simulink subsystem "DiffSwerveChassisSimulation"  (R2022a)
settings: Solver=VariableStepAuto  StartTime=0.0  StopTime=10.0  RelTol=1e-3
values from neighbouring files (symbols this model uses):
  chassis = struct(     'M_inv', M_inv,     'M', M,     'num_modules', num_modules,     'module_locations', module_locations )    [GetDiffSwerveChassis.m]
undefined symbols (not defined in the file or in its folder): theta0, x0, y0
settings Model: Creator=woz4t  LastModifiedBy=woz4t

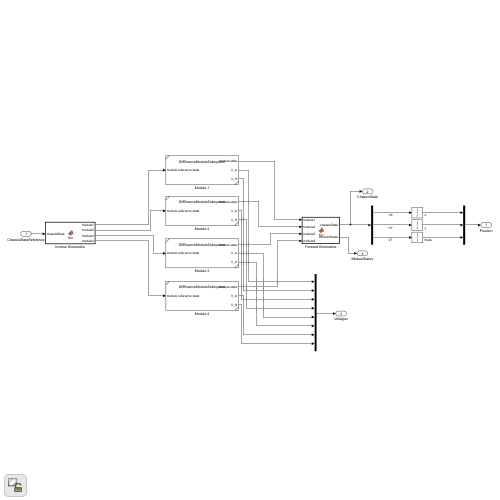
[thumbnail: Simulink's stored preview of the top-level diagram]
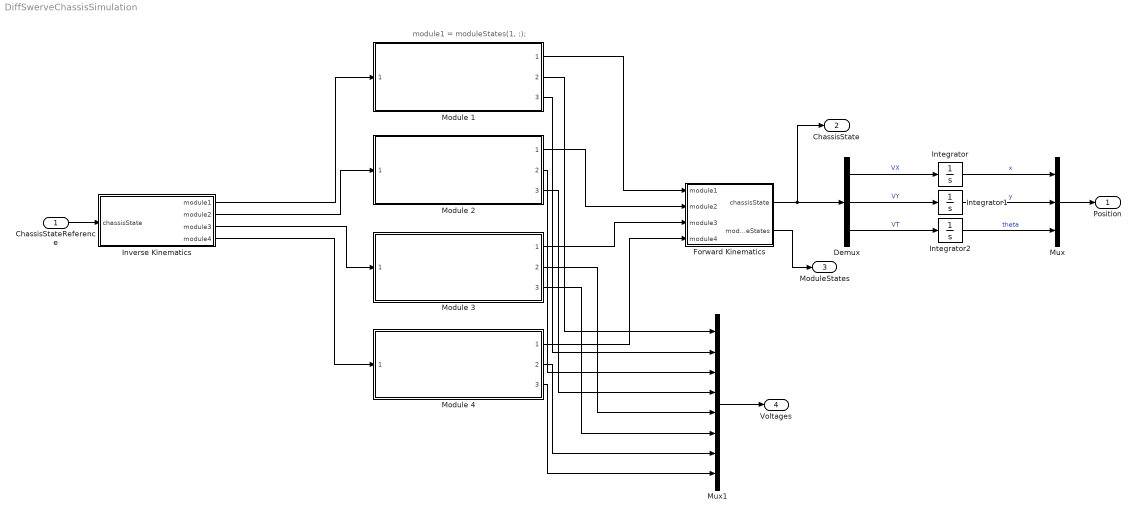
== system DiffSwerveChassisSimulation ==
  note: module1 = moduleStates(1, :);
  ChassisStateReference : Inport
  Demux : Demux  Outputs=3
  Forward Kinematics : MATLAB Function  TreatAsAtomicUnit=on  mask{M=chassis.M}
  Integrator : Integrator  InitialCondition=x0
  Integrator1 : Integrator  InitialCondition=y0
  Integrator2 : Integrator  InitialCondition=theta0
  Inverse Kinematics : MATLAB Function  TreatAsAtomicUnit=on  mask{M_inv=chassis.M_inv, num_modules=chassis.num_modules}
  Module {1..4} (4 alike) : Subsystem  ReferencedSubsystem=DiffSwerveModuleSubsystem
  Mux : Mux  Inputs=3
  Mux1 : Mux  Inputs=8
  Position : Outport
  ChassisState : Outport  Port=2
  ModuleStates : Outport  Port=3
  Voltages : Outport  Port=4
  wires:
  Integrator/1 -> Mux/1  "x"
  Forward Kinematics/1(chassisState) -> Demux/1, ChassisState/1
  Module 1/1 -> Forward Kinematics/1(module1)
  Inverse Kinematics/3(module3) -> Module 3/1
  Integrator2/1 -> Mux/3  "theta"
  Inverse Kinematics/4(module4) -> Module 4/1
  Demux/1 -> Integrator/1  "VX"
  Demux/2 -> Integrator1/1  "VY"
  ChassisStateReference/1 -> Inverse Kinematics/1(chassisState)
  Inverse Kinematics/2(module2) -> Module 2/1
  Module 3/1 -> Forward Kinematics/3(module3)
  Demux/3 -> Integrator2/1  "VT"
  Inverse Kinematics/1(module1) -> Module 1/1
  Integrator1/1 -> Mux/2  "y"
  Module 4/1 -> Forward Kinematics/4(module4)
  Module 2/1 -> Forward Kinematics/2(module2)
  Mux/1 -> Position/1
  Forward Kinematics/2(moduleStates) -> ModuleStates/1
  Module 1/2 -> Mux1/1
  Module 1/3 -> Mux1/2
  Module 2/2 -> Mux1/3
  Module 2/3 -> Mux1/4
  Module 3/2 -> Mux1/5
  Module 3/3 -> Mux1/6
  Module 4/2 -> Mux1/7
  Module 4/3 -> Mux1/8
  Mux1/1 -> Voltages/1

== matlab function DiffSwerveChassisSimulation/Forward Kinematics ==
  data: module1 input; chassisState output; module2 input; module3 input; module4 input; M parameter; moduleStates output
function [chassisState, moduleStates] = fcn(module1, module2, module3, module4, M)

moduleStates = zeros(4, 3);
moduleStates(1, :) = module1';
moduleStates(2, :) = module2';
moduleStates(3, :) = module3';
moduleStates(4, :) = module4';

chassisState = ChassisForwardKinematics(M, moduleStates);

== matlab function DiffSwerveChassisSimulation/Inverse Kinematics ==
  data: module1 output; chassisState input size=3; module2 output; module3 output; num_modules parameter size=1; M_inv parameter; module4 output
function [module1, module2, module3, module4] = fcn(chassisState, num_modules, M_inv)

moduleStates = ChassisInverseKinematics(M_inv, num_modules, chassisState);
module1 = moduleStates(1, :)';
module2 = moduleStates(2, :)';
module3 = moduleStates(3, :)';
module4 = moduleStates(4, :)';
% azimuth = chassisState(1);
% azimuth_velocity = chassisState(2);
% wheel_velocity = chassisState(3);
